simulink model "Q2"  (R2018b)
settings: Solver=VariableStepAuto  StartTime=0.0  StopTime=250  RelTol=1e-3
values from neighbouring files (symbols this model uses):
  n = 5    [Q2Code.m]
undefined symbols (not defined in the file or in its folder): m
settings Model: Creator=lenovo  LastModifiedBy=lenovo

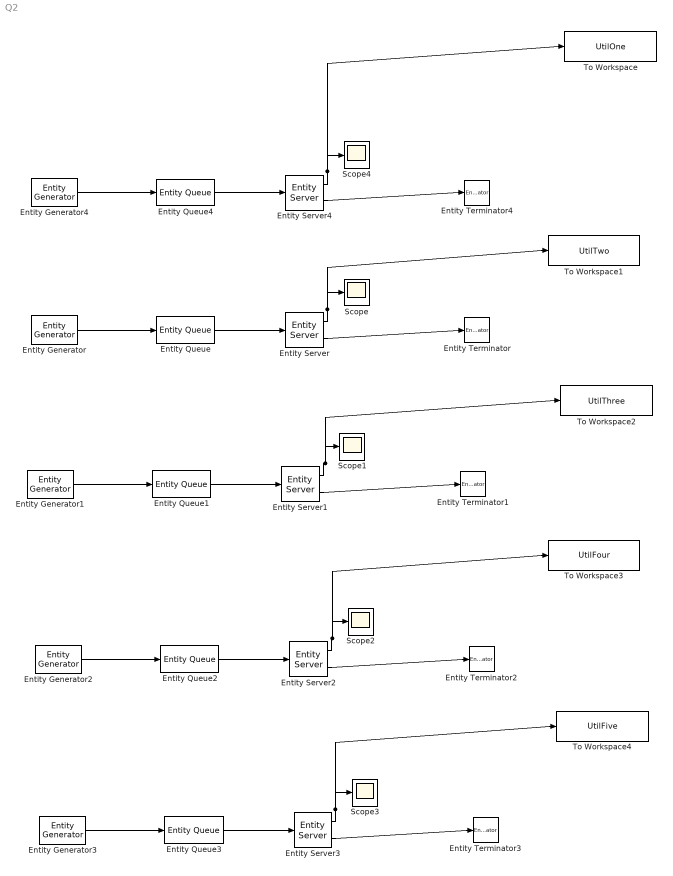
== system Q2 ==
  Entity Generator : EntityGenerator  OutputPortMessageModes=m  TimeSource=MATLAB action  Period=5  IntergenerationTimeAction=|  EntityType=Structured  EntityTypeName=Entity
      | persistent rngInit;
      | if isempty(rngInit)
      |     seed = 71239;
      |     rng(seed);
      |     rngInit = true;
      | end
      | persistent generatedNum;
      | if isempty(generatedNum)
      |    generatedNum = 1;
      | end 
      | if generatedNum <= 100
      |     % Pattern: Exponential distribution
      |     mu = 2;
      |     dt = -mu * log(1 - rand());
      | else
      |     dt = inf;
      | end
      | generatedNum = generatedNum + 1;
  Entity Generator1 : EntityGenerator  OutputPortMessageModes=m  TimeSource=MATLAB action  Period=5  IntergenerationTimeAction=|  EntityType=Structured  EntityTypeName=Entity
      | persistent rngInit;
      | if isempty(rngInit)
      |     seed = 12653;
      |     rng(seed);
      |     rngInit = true;
      | end
      | persistent generatedNum;
      | if isempty(generatedNum)
      |    generatedNum = 1;
      | end 
      | if generatedNum <= 100
      |     % Pattern: Exponential distribution
      |     mu = 2;
      |     dt = -mu * log(1 - rand());
      | else
      |     dt = inf;
      | end
      | generatedNum = generatedNum + 1;
  Entity Generator2 : EntityGenerator  OutputPortMessageModes=m  TimeSource=MATLAB action  Period=5  IntergenerationTimeAction=|  EntityType=Structured  EntityTypeName=Entity
      | persistent rngInit;
      | if isempty(rngInit)
      |     seed = 19823;
      |     rng(seed);
      |     rngInit = true;
      | end
      | persistent generatedNum;
      | if isempty(generatedNum)
      |    generatedNum = 1;
      | end 
      | if generatedNum <= 100
      |     % Pattern: Exponential distribution
      |     mu = 2;
      |     dt = -mu * log(1 - rand());
      | else
      |     dt = inf;
      | end
      | generatedNum = generatedNum + 1;
  Entity Generator3 : EntityGenerator  OutputPortMessageModes=m  TimeSource=MATLAB action  Period=5  IntergenerationTimeAction=|  EntityType=Structured  EntityTypeName=Entity
      | persistent rngInit;
      | if isempty(rngInit)
      |     seed = 23784;
      |     rng(seed);
      |     rngInit = true;
      | end
      | persistent generatedNum;
      | if isempty(generatedNum)
      |    generatedNum = 1;
      | end 
      | if generatedNum <= 100
      |     % Pattern: Exponential distribution
      |     mu = 2;
      |     dt = -mu * log(1 - rand());
      | else
      |     dt = inf;
      | end
      | generatedNum = generatedNum + 1;
  Entity Generator4 : EntityGenerator  OutputPortMessageModes=m  TimeSource=MATLAB action  Period=5  IntergenerationTimeAction=|  EntityType=Structured  EntityTypeName=Entity
      | persistent rngInit;
      | if isempty(rngInit)
      |     seed = 83721;
      |     rng(seed);
      |     rngInit = true;
      | end
      | persistent generatedNum;
      | if isempty(generatedNum)
      |    generatedNum = 1;
      | end 
      | if generatedNum <= 100
      |     % Pattern: Exponential distribution
      |     mu = 2;
      |     dt = -mu * log(1 - rand());
      | else
      |     dt = inf;
      | end
      | generatedNum = generatedNum + 1
  Entity Queue{,1..4} (5 alike) : EntityQueue  InputPortMessageModes=m  OutputPortMessageModes=m  Capacity=inf
      settings: OutputPortMap=o5
  Entity Server : EntityServer  InputPortMessageModes=m  OutputPortMessageModes=n,m  Capacity=1  ServiceTimeSource=MATLAB action  ServiceTimeAttributeName=Attribute1  ServiceTimeAction=|  Utilization=on
      | persistent rngInit;
      | if isempty(rngInit)
      |     seed = 18273;
      |     rng(seed);
      |     rngInit = true;
      | end
      | 
      | % Pattern: Gaussian (normal) distribution
      | % m: Mean, d: Standard deviation
      | m = 3; d = 0.04;
      | dt = m + d * randn;
      settings: OutputPortMap=o5,o9
  Entity Server1 : EntityServer  InputPortMessageModes=m  OutputPortMessageModes=n,m  Capacity=1  ServiceTimeSource=MATLAB action  ServiceTimeAttributeName=Attribute1  ServiceTimeAction=|  Utilization=on
      | persistent rngInit;
      | if isempty(rngInit)
      |     seed = 23658;
      |     rng(seed);
      |     rngInit = true;
      | end
      | 
      | % Pattern: Gaussian (normal) distribution
      | % m: Mean, d: Standard deviation
      | m = 3; d = 0.04;
      | dt = m + d * randn;
      settings: OutputPortMap=o5,o9
  Entity Server2 : EntityServer  InputPortMessageModes=m  OutputPortMessageModes=n,m  Capacity=1  ServiceTimeSource=MATLAB action  ServiceTimeAttributeName=Attribute1  ServiceTimeAction=|  Utilization=on
      | persistent rngInit;
      | if isempty(rngInit)
      |     seed = 71235;
      |     rng(seed);
      |     rngInit = true;
      | end
      | 
      | % Pattern: Gaussian (normal) distribution
      | % m: Mean, d: Standard deviation
      | m = 3; d = 0.04;
      | dt = m + d * randn;
      settings: OutputPortMap=o5,o9
  Entity Server3 : EntityServer  InputPortMessageModes=m  OutputPortMessageModes=n,m  Capacity=1  ServiceTimeSource=MATLAB action  ServiceTimeAttributeName=Attribute1  ServiceTimeAction=|  Utilization=on
      | persistent rngInit;
      | if isempty(rngInit)
      |     seed = 91283;
      |     rng(seed);
      |     rngInit = true;
      | end
      | 
      | % Pattern: Gaussian (normal) distribution
      | % m: Mean, d: Standard deviation
      | m = 3; d = 0.04;
      | dt = m + d * randn;
      settings: OutputPortMap=o5,o9
  Entity Server4 : EntityServer  InputPortMessageModes=m  OutputPortMessageModes=n,m  Capacity=1  ServiceTimeSource=MATLAB action  ServiceTimeAttributeName=Attribute1  ServiceTimeAction=|  Utilization=on
      | persistent rngInit;
      | if isempty(rngInit)
      |     seed = 12345;
      |     rng(seed);
      |     rngInit = true;
      | end
      | 
      | % Pattern: Gaussian (normal) distribution
      | % m: Mean, d: Standard deviation
      | m = 3; d = 0.04;
      | dt = m + d * randn;
      settings: OutputPortMap=o5,o9
  Entity Terminator{,1..4} (5 alike) : EntityTerminator  InputPortMessageModes=m
  Scope{,1..4} (5 alike) : Scope
  To Workspace : ToWorkspace  VariableName=UtilOne  SampleTime=-1
  To Workspace1 : ToWorkspace  VariableName=UtilTwo  SampleTime=-1
  To Workspace2 : ToWorkspace  VariableName=UtilThree  SampleTime=-1
  To Workspace3 : ToWorkspace  VariableName=UtilFour  SampleTime=-1
  To Workspace4 : ToWorkspace  VariableName=UtilFive  SampleTime=-1
  wires:
  Entity Server/1 -> To Workspace1/1, Scope/1
  Entity Generator/1 -> Entity Queue/1
  Entity Server/2 -> Entity Terminator/1
  Entity Queue/1 -> Entity Server/1
  Entity Server1/2 -> Entity Terminator1/1
  Entity Queue1/1 -> Entity Server1/1
  Entity Generator1/1 -> Entity Queue1/1
  Entity Server1/1 -> To Workspace2/1, Scope1/1
  Entity Server2/2 -> Entity Terminator2/1
  Entity Queue2/1 -> Entity Server2/1
  Entity Generator2/1 -> Entity Queue2/1
  Entity Server2/1 -> To Workspace3/1, Scope2/1
  Entity Server3/2 -> Entity Terminator3/1
  Entity Queue3/1 -> Entity Server3/1
  Entity Generator3/1 -> Entity Queue3/1
  Entity Server4/2 -> Entity Terminator4/1
  Entity Queue4/1 -> Entity Server4/1
  Entity Generator4/1 -> Entity Queue4/1
  Entity Server4/1 -> To Workspace/1, Scope4/1
  Entity Server3/1 -> To Workspace4/1, Scope3/1
